simulink model "zad_4_sch_stalowartosciowa"  (R2022b)
settings: Solver=FixedStepAuto  StartTime=0.0  StopTime=5  FixedStep=0.0001  RelTol=1e-3
values from neighbouring files (symbols this model uses):
  a21 = 1/(2*m)*x30^2*FemP1/FemP2^2*exp(-x10/FemP2)    [zad_4.m]
  a23 = -1/(m)*x30*FemP1/FemP2*exp(-x10/FemP2)    [zad_4.m]
  a31 = 1/f1*exp(x10/f2)*(ki*u10+ci-x30)    [zad_4.m]
  a33 = -f2/f1*exp(x10/f2)    [zad_4.m]
  b31 = ki*f2/f1*exp(x10/f2)    [zad_4.m]
  g = 9.81    [zad_4.m]
  k = -place(A, B(:,1), -s)    [zad_4.m]
  u0 = -(a31*x1+a33*x3)/b31    [zad_4.m]
  x1 = .008    (= 0.008)    [zad_4.m]
  x2 = 0    [zad_4.m]
  x3 = -(a21*x1+g)/a23    [zad_4.m]
  xd = d-bd    (= 0.0192)    [zad_4.m]
settings Model: Creator=AgraWoodAdmin  LastModifiedBy=AgraWoodAdmin
settings DebuggingCC: UnconnectedInputMsg=warning  UnconnectedOutputMsg=warning  UnconnectedLineMsg=warning
settings ModelReferenceCC: EnableRefExpFcnMdlSchedulingChecks=on
settings RTWCC: DLArmComputeVersion=19.05

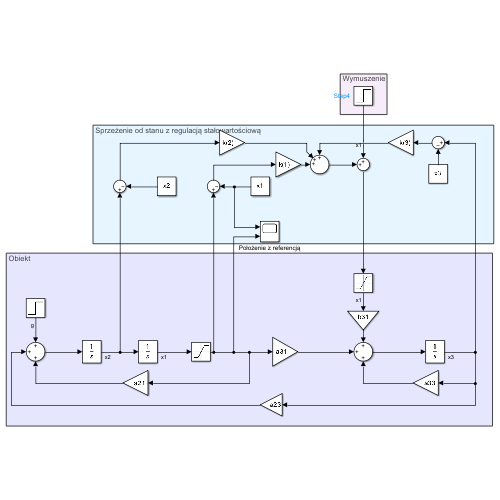
[thumbnail: Simulink's stored preview of the top-level diagram]
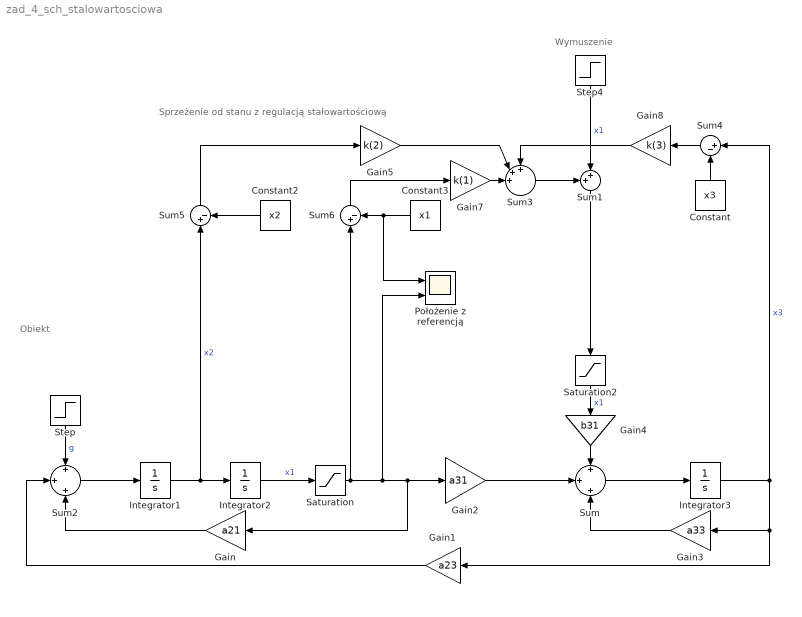
== system zad_4_sch_stalowartosciowa ==
  note: Sprzeżenie od stanu z regulacją stałowartościową
  note: Obiekt
  note: Wymuszenie
  Constant : Constant  Value=x3
  Constant2 : Constant  Value=x2
  Constant3 : Constant  Value=x1
  Gain : Gain  Gain=a21
  Gain1 : Gain  Gain=a23
  Gain2 : Gain  Gain=a31
  Gain3 : Gain  Gain=a33
  Gain4 : Gain  Gain=b31
  Gain5 : Gain  Gain=k(2)
  Gain7 : Gain  Gain=k(1)
  Gain8 : Gain  Gain=k(3)
  Integrator1 : Integrator
  Integrator2 : Integrator  InitialCondition=xd
  Integrator3 : Integrator
  Położenie z referencją : Scope  NumInputPorts=2
  Saturation : Saturate  UpperLimit=xd  LowerLimit=0
  Saturation2 : Saturate  UpperLimit=1  LowerLimit=0
  Step : Step  Time=0  After=g  SampleTime=0
  Step4 : Step  Time=0  After=u0  SampleTime=0
  Sum : Sum  Inputs=+|+|+
  Sum1 : Sum  Inputs=++|
  Sum2 : Sum  Inputs=+|+|+
  Sum3 : Sum  Inputs=+++||
  Sum4 : Sum  Inputs=|+-
  Sum5 : Sum  Inputs=|+-
  Sum6 : Sum  Inputs=|+-
  wires:
  Sum2/1 -> Integrator1/1
  Sum/1 -> Integrator3/1
  Integrator1/1 -> Integrator2/1, Sum5/1  "x2"
  Integrator3/1 -> Gain1/1, Gain3/1, Sum4/1  "x3"
  Gain/1 -> Sum2/3
  Gain1/1 -> Sum2/2
  Gain3/1 -> Sum/3
  Gain4/1 -> Sum/1
  Step/1 -> Sum2/1  "g"
  Saturation/1 -> Gain2/1, Gain/1, Położenie z referencją/2, Sum6/1
  Step4/1 -> Sum1/2  "x1"
  Sum1/1 -> Saturation2/1
  Gain7/1 -> Sum3/3
  Gain5/1 -> Sum3/2
  Gain8/1 -> Sum3/1
  Sum3/1 -> Sum1/1
  Sum4/1 -> Gain8/1
  Constant/1 -> Sum4/2
  Sum5/1 -> Gain5/1
  Constant2/1 -> Sum5/2
  Sum6/1 -> Gain7/1
  Constant3/1 -> Położenie z referencją/1, Sum6/2
  Saturation2/1 -> Gain4/1  "x1"
  Integrator2/1 -> Saturation/1  "x1"
  Gain2/1 -> Sum/2
